simulink model "fir_simulink"  (Simulink 7.0)
settings: Solver=FixedStepDiscrete  SolverMode=SingleTasking  StartTime=0.0  StopTime=500*Tsamp  RelTol=1e-3
PreLoadFcn:
  | init
InitFcn:
  | %% DSPBuilder Start
  | alt_dspbuilder_update_model(bdroot)
  | %% DSPBuilder End
values from neighbouring files (symbols this model uses):
  Tsamp = 1    [init.m]
undefined symbols (not defined in the file or in its folder): DSPBuilder_fir_simulink_import, final_add, fir_vhdl, four_mult_add
libraries: allblocks_alteradspbuilder2 x7, simulink x1
settings Model: Creator=gnixon  LastModifiedBy=gdesilva
settings DebuggingCC: SaveWithParameterizedLinksMsg=none  SignalResolutionControl=TryResolveAllWithWarning  MultiTaskDSMMsg=warning  MultiTaskCondExecSysMsg=none
settings RTWCC: IncludeERTFirstTime=on
settings GRTTargetCC: TargetFcnLib=ansi_tfl_tmw.mat

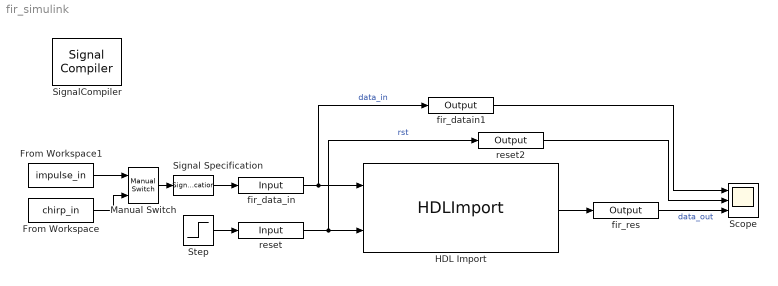
== system fir_simulink ==
  From Workspace : FromWorkspace  VariableName=chirp_in  SampleTime=Tsamp
  From Workspace1 : FromWorkspace  VariableName=impulse_in  SampleTime=Tsamp
  HDL Import : allblocks_alteradspbuilder2/HDLImport  entityName=fir_vhdl_import  inNames=data_in sclr  inBwls=16 1  inBwrs="0  0"  inTypes=s b  inDelayed="0  0"  outNames=data_out  outBwls=33  outBwrs=0  outTypes=s  xmlmapfile=q:\altera\quartus\dsp_builder\lib\SimgenCMap.xml  vofile=DSPBuilder_fir_simulink_import/fir_vhdl.vo  src_file=four_mult_add.vhd;final_add.vhd;fir_vhdl.vhd;  TopLevelName=fir_vhdl  UseQPF=0  n_input_port=2  n_output_port=1  array_clocks=clock  use_systemC_model=off  is_megacore=off  use_dynamic_feedthrough_data=off  use_alphabetical_port_ordering=on  allowFloatingPointOverride=off
  Manual Switch : simulink/Signal Routing/Manual Switch  SystemSampleTime=-1  sw=0  action=0  varsize=off
  Scope : Scope  NumInputPorts=3
      settings: YMin=-40000~-1~-1  YMax=40000~1~1
  Signal Specification : SignalSpecification  SampleTime=Tsamp  OutDataType=sfix(16)  OutScaling=2^0
  SignalCompiler : allblocks_alteradspbuilder2/Signal Compiler  DeviceFamily=Stratix III  DeviceName=AUTO  EnableSignalTap=off  SignalTapDepth=128  UseBoardBlock=off  StpUseDefaultClock=on  StpClock=clock  ExportDir=.
  Step : Step  Time=3  Before=1  After=0  SampleTime=1
  fir_data_in : allblocks_alteradspbuilder2/Input  iofile=D:\spr\286893\BlackBox\update\HDLImport\HDLImport\tb_fir_simulink\fir%5Fsimulink_fir%5Fdata%5Fin.salt  BusType=Signed Integer  bwl=16  bwr=0  SpecifyClock=off  PORTTYPE=Input  externalType=Inferred  allowFloatingPointOverride=on  logOutputs=off
  fir_datain1 : allblocks_alteradspbuilder2/Output  iofile=D:\spr\286893\BlackBox\update\HDLImport\HDLImport\tb_fir_simulink\fir%5Fsimulink_fir%5Fdatain1.capture  BusType=Signed Integer  bwl=16  bwr=0  externalType=Inferred  PORTTYPE=Output  allowFloatingPointOverride=on  logOutputs=off
  fir_res : allblocks_alteradspbuilder2/Output  iofile=D:\spr\286893\BlackBox\update\HDLImport\HDLImport\tb_fir_simulink\fir%5Fsimulink_fir%5Fres.capture  BusType=Signed Integer  bwl=33  bwr=0  externalType=Inferred  PORTTYPE=Output  allowFloatingPointOverride=on  logOutputs=off
  reset : allblocks_alteradspbuilder2/Input  iofile=D:\spr\286893\BlackBox\update\HDLImport\HDLImport\tb_fir_simulink\fir%5Fsimulink_reset.salt  BusType=Single Bit  bwl=1  bwr=0  SpecifyClock=off  PORTTYPE=Input  externalType=Inferred  allowFloatingPointOverride=on  logOutputs=off
  reset2 : allblocks_alteradspbuilder2/Output  iofile=D:\spr\286893\BlackBox\update\HDLImport\HDLImport\tb_fir_simulink\fir%5Fsimulink_reset2.capture  BusType=Single Bit  bwl=16  bwr=0  externalType=Inferred  PORTTYPE=Output  allowFloatingPointOverride=on  logOutputs=off
  wires:
  fir_data_in/1 -> HDL Import/1, fir_datain1/1  "data_in"
  Signal Specification/1 -> fir_data_in/1
  reset/1 -> HDL Import/2, reset2/1  "rst"
  HDL Import/1 -> fir_res/1
  Step/1 -> reset/1
  fir_res/1 -> Scope/3  "data_out"
  Manual Switch/1 -> Signal Specification/1
  From Workspace1/1 -> Manual Switch/1
  From Workspace/1 -> Manual Switch/2
  fir_datain1/1 -> Scope/1
  reset2/1 -> Scope/2
